simulink model "esa"  (R2018a)
settings: Solver=VariableStepAuto  StartTime=0.0  StopTime=10.0  RelTol=1e-3
values from neighbouring files (symbols this model uses):
  wm = imread('Capture2.png')    [datahide.m]    (also in extractdata.m = reshape(wm_str, im_sz , im_sz))
libraries: dspvision x2, dspsnks4 x1, visionsources x1
settings Model: Creator=The Phantom Stranger  LastModifiedBy=The Phantom Stranger

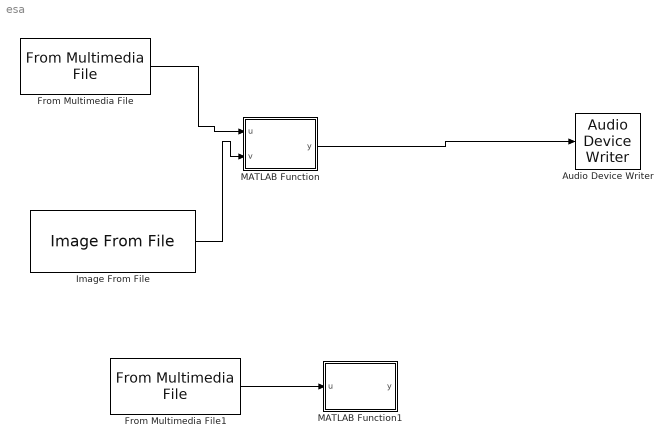
== system esa ==
  Audio Device Writer : dspsnks4/Audio Device Writer  Driver=DirectSound  Device=Default  InheritSampleRate=on  SampleRate=44100  BitDepth=16-bit integer  BufferSize=4096  NumBuffers=10  DefaultOutputChannelMapping=on  OutputChannelMapping=1:2  OutputNumUnderrunSamples=off  DriverIdx=1  DeviceWarnFlag=''
  From Multimedia File : dspvision/From Multimedia File  inputFilename=C:\Users\HP\Downloads\Telegram Desktop\wm\BabyElephantWalk60.wav  loop=on  numPlays=inf  outputStreams=Audio only  videoDataType=single  audioDataType=double  inheritSampleTime=on  userDefinedSampleTime=1/30  noAudioOutput=off  isIntensityVideo=off  fourcc=RGB  colorVideoFormat=Separate color signals  outputEOF=off  dataOrg=Column-major  audioFrameSize=1024  computeAudioFrameSize=off  outSamplingMode=Sample based
      settings: SourceProductBaseCode=VP
  From Multimedia File1 : dspvision/From Multimedia File  inputFilename=C:\wm\NEWMSG.wav  loop=on  numPlays=inf  outputStreams=Audio only  videoDataType=single  audioDataType=double  inheritSampleTime=on  userDefinedSampleTime=1/30  noAudioOutput=off  isIntensityVideo=off  fourcc=RGB  colorVideoFormat=Separate color signals  outputEOF=off  dataOrg=Column-major  audioFrameSize=1024  computeAudioFrameSize=off  outSamplingMode=Sample based
      settings: SourceProductBaseCode=VP
  Image From File : visionsources/Image From File  Tag=vipblks_nd  FileName=C:\Users\HP\Downloads\Telegram Desktop\done deal\done deal\watermark.png  imagePorts=One multidimensional signal  Ts=inf  ImageDataType=Inherit from input image  Signed=on  WordLength=16  sdImageDataType=uint(8)  FractionLengthMode=User-defined  FractionLength=15  OutPortLabels=R|G|B
      settings: SourceProductName=Computer Vision System Toolbox
  MATLAB Function : MATLAB Function  TreatAsAtomicUnit=on
  MATLAB Function1 : MATLAB Function  TreatAsAtomicUnit=on
  wires:
  From Multimedia File/1 -> MATLAB Function/1(u)
  Image From File/1 -> MATLAB Function/2(v)
  MATLAB Function/1(y) -> Audio Device Writer/1
  From Multimedia File1/1 -> MATLAB Function1/1(u)

== matlab function esa/MATLAB Function1 ==
  data: u input; y output
function y = fcn(u)
%Extracting hidden image from water marked audio signal
clc
clear
close all 
wm_sz     = 20000;                        % watermark size
px_sz     = wm_sz/8;                      % number of pixels
im_sz     = sqrt(px_sz);                  % image size
msg_new  = audioread ('NEWMSG.wav');   % new (watermarked) host signal
msg_new  = uint8(255*(msg_new + 0.5));  % double [-0.5 +0.5] to 'uint8' [0 255]

% prepare host
msg_bin  = dec2bin(msg_new, 8);         % binary host [n 8]

% extract watermark
wm_bin_str = msg_bin(1:wm_sz, 8);
wm_bin    = reshape(wm_bin_str, px_sz , 8);
wm_str    = zeros(px_sz, 1, 'uint8');

for i     = 1:px_sz                        % extract water mark from the first plane of host               
    wm_str(i, :) = bin2dec(wm_bin(i, :));      % Least Significant Bit (LSB)
end

wm  = reshape(wm_str, im_sz , im_sz);

% show image
imshow(wm);
%imwrite(wm,map,'kal.png');

y = u;

== matlab function esa/MATLAB Function ==
  data: y output; u input; v input
function y = fcn(u,v)
% hiding image data in audio signal AKA watermarking
%importing audio data from fi
[msg, f] = audioread (u);   %message variable msg
msg      = uint8(255*(msg + 0.5));  % double to 'uint8' 
wm        = imread(v);  %  Image data to be hidden aka watermark 
[r, c]    = size(wm);                 % watermark size
wm_ln      = length(wm(:))*8;          % watermark length
% watermark size checking
if length(msg) < (length(wm(:))*8)
    disp('The audio file and the image file and disproportinate please select larger audio file or smaller image file')
else
%watermarking    
% prepare host
msg_bin  = dec2bin(msg, 8);         
% prepare watermark   
wm_bin    = dec2bin(wm(:), 8);        
wm_str    = zeros(wm_ln, 1);           

for j = 1:8                           
    for i = 1:length(wm(:))
        ind   = (j-1)*length(wm(:)) + i;
        wm_str(ind, 1) = str2double(wm_bin(i, j));
    end
end
% insert watermark into the host

for i     = 1:wm_ln                   % insert water mark into the first plane of host               
msg_bin(i, 8) = dec2bin(wm_str(i)); % Least Significant Bit (LSB)
end 
% watermarked host
msg_new  = bin2dec(msg_bin);       
msg_new  = (double(msg_new)/255 - 0.5);   % 'uint8' to double
% save the watermarked message to "newmsg.wav" file
audiowrite(y, msg_new, f)     
end
